simulink model "multi_rotor_sim"  (R2023b)
settings: Solver=ode4  StartTime=0.0  StopTime=inf  FixedStep=ST  RelTol=1e-3
values from neighbouring files (symbols this model uses):
  a0 = 0    [parameters.m]
  ASLOPE = 5.9    [parameters.m]
  Ax = 0.023    [parameters.m]
  Ay = 0.023    [parameters.m]
  Az = 0.106    [parameters.m]
  BLADES = 2    [parameters.m]
  BLCG = 0    [parameters.m]
  BLCP = 0    [parameters.m]
  BLH1 = b*sind(30)    [parameters.m]
  BLH2 = b    (= 0.275)    [parameters.m]
  BLH3 = b*sind(30)    [parameters.m]
  BLH4 = -b*sind(30)    [parameters.m]
  BLH5 = -b    (= -0.275)    [parameters.m]
  BLH6 = -b*sind(30)    [parameters.m]
  chi1 = 1    [parameters.m]
  chi2 = -1    [parameters.m]
  chi3 = 1    [parameters.m]
  chi4 = -1    [parameters.m]
  chi5 = 1    [parameters.m]
  chi6 = -1    [parameters.m]
  CHORD = 17.55e-3    (= 0.01755)    [parameters.m]
  CHORD75 = 21e-3    (= 0.021)    [parameters.m]
  dyn_viscosity = 17.89e-6    (= 1.789e-05)    [parameters.m]
  g0 = 9.80665    [parameters.m]
  href = 0    [parameters.m]
  k_ind = 1.35    [parameters.m]
  k_Omega = 14.92    [parameters.m]
  latref = 44.200626    [parameters.m]
  lonref = 12.063822    [parameters.m]
  m = 2.15    [parameters.m]
  MC_ATT_PITCH = 45*pi/180    (= 0.785398163397)    [parameters.m]
  MC_ATT_ROLL = 45*pi/180    (= 0.785398163397)    [parameters.m]
  MC_PITCH_P = 2    [parameters.m]
  MC_PITCHRATE_D = 0    [parameters.m]
  MC_PITCHRATE_I = 0.05    [parameters.m]
  MC_PITCHRATE_P = 0.09*3    (= 0.27)    [parameters.m]
  MC_RATE_PITCH = 500*pi/180    (= 8.72664625997)    [parameters.m]
  MC_RATE_ROLL = 500*pi/180    (= 8.72664625997)    [parameters.m]
  MC_RATE_YAW = 300*pi/180    (= 5.23598775598)    [parameters.m]
  MC_ROLL_P = 2    [parameters.m]
  MC_ROLLRATE_D = 0    [parameters.m]
  MC_ROLLRATE_I = 0.05    [parameters.m]
  MC_ROLLRATE_P = 0.09*3    (= 0.27)    [parameters.m]
  MC_VEL_FWD = 15    [parameters.m]
  MC_VEL_FWD_OPT = 0.5    [parameters.m]
  MC_VEL_LAT = 15    [parameters.m]
  MC_VEL_LAT_OPT = 0.5    [parameters.m]
  MC_VEL_VERT = 15    [parameters.m]
  MC_YAW_P = 0.55    [parameters.m]
  MC_YAWRATE_D = 0.05    [parameters.m]
  MC_YAWRATE_I = 0.02    [parameters.m]
  MC_YAWRATE_P = 0.15*3    (= 0.45)    [parameters.m]
  MPC_XY_VEL_D_ACC = 0.6    [parameters.m]
  MPC_XY_VEL_I_ACC = 0.8    [parameters.m]
  MPC_XY_VEL_P_ACC = 1.7    [parameters.m]
  MPC_Z_VEL_D_ACC = 0    [parameters.m]
  MPC_Z_VEL_I_ACC = 2    [parameters.m]
  MPC_Z_VEL_P_ACC = 4    [parameters.m]
  n = 0.6359    [parameters.m]
  p00 = 7.145e-2    (= 0.07145)    [parameters.m]
  p01 = 0.4377    [parameters.m]
  p02 = -10.13    [parameters.m]
  p10 = 1.259e-3    (= 0.001259)    [parameters.m]
  p11 = 1.284e-3    (= 0.001284)    [parameters.m]
  p20 = -7.513e-7    (= -7.513e-07)    [parameters.m]
  PWM_hover = (PWM_idle+PWM_max)/2    (= 1550)    [parameters.m]
  PWM_idle = 1100    [parameters.m]
  PWM_max = 2000    [parameters.m]
  ROTOR = 4*0.0254    (= 0.1016)    [parameters.m]
  ST = 0.01    [parameters.m]
  STACG = 0    [parameters.m]
  STACP = 0    [parameters.m]
  STAH1 = -b*cosd(30)    [parameters.m]
  STAH2 = 0    [parameters.m]
  STAH3 = b*cosd(30)    [parameters.m]
  STAH4 = b*cosd(30)    [parameters.m]
  STAH5 = 0    [parameters.m]
  STAH6 = -b*cosd(30)    [parameters.m]
  TERMINAL_SPEED = 0.5    [parameters.m]
  Theta0 = 45*pi/180    (= 0.785398163397)    [parameters.m]
  THETT = -38.0973*pi/180    (= -0.66492332112)    [parameters.m]
  wind_rate = [ 0 0 0 ]'    [parameters.m]
  wind_velocity_e = [ 0 0 0 ]'    [parameters.m]
  WLCG = -0.02    [parameters.m]
  WLCP = -0.08    [parameters.m]
  WLH1 = 32e-3    (= 0.032)    [parameters.m]
  WLH2 = 32e-3    (= 0.032)    [parameters.m]
  WLH3 = 32e-3    (= 0.032)    [parameters.m]
  WLH4 = 32e-3    (= 0.032)    [parameters.m]
  WLH5 = 32e-3    (= 0.032)    [parameters.m]
  WLH6 = 32e-3    (= 0.032)    [parameters.m]
undefined symbols (not defined in the file or in its folder): Earth, WGS84, X, Y, Z
libraries: sm_lib x258, slpidlib x36, nesl_utility x15, sharedtransform x13, aerolibutil x4, aerolibanimutils x3, sharedutil x2, sim3dlib x1, uavsim3dlib x1, shared6dof x1, aerolibtransform2 x1, aerolibatmos2 x1
(part 1 of 11)
settings Model: Creator=Francesco Sessini  LastModifiedBy=fra62

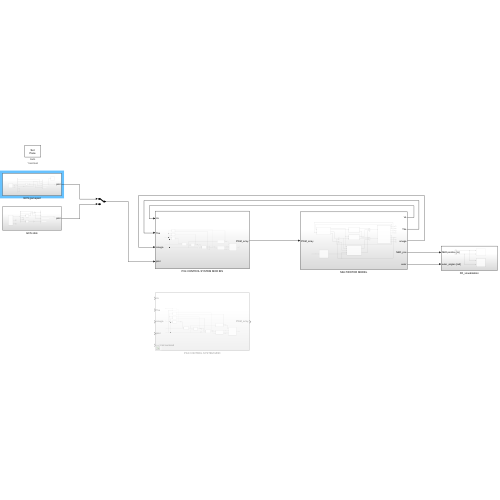
[thumbnail: Simulink's stored preview of the top-level diagram]
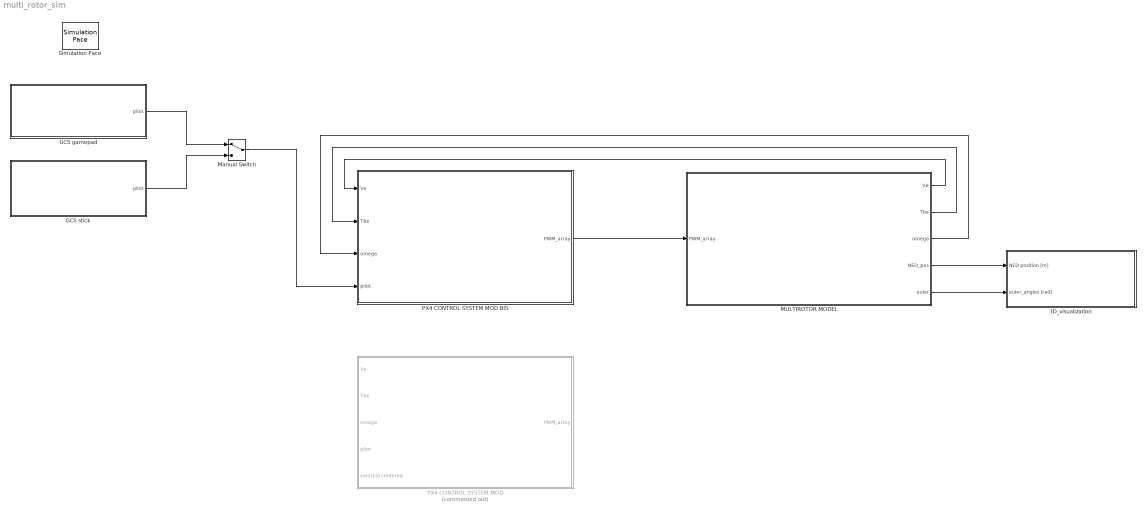
== system multi_rotor_sim ==
  3D_visualization : Subsystem
  GCS gamepad : Subsystem
  GCS stick : Subsystem
  MULTIROTOR MODEL : Subsystem
  Manual Switch : ManualSwitch
  PX4 CONTROL SYSTEM MOD : Subsystem  Commented=on
  PX4 CONTROL SYSTEM MOD BIS : Subsystem
  Simulation Pace : aerolibanimutils/Simulation Pace  SimulationPace=1  SleepMode=Auto  OutputPaceError=off  SampleTime=ST
  wires:
  PX4 CONTROL SYSTEM MOD BIS/1(PWM_array) -> MULTIROTOR MODEL/1(PWM_array)
  MULTIROTOR MODEL/1(Ve) -> PX4 CONTROL SYSTEM MOD BIS/1(Ve)
  MULTIROTOR MODEL/2(Tbe) -> PX4 CONTROL SYSTEM MOD BIS/2(Tbe)
  MULTIROTOR MODEL/3(omega) -> PX4 CONTROL SYSTEM MOD BIS/3(omega)
  Manual Switch/1 -> PX4 CONTROL SYSTEM MOD BIS/4(pilot)
  GCS stick/1(pilot) -> Manual Switch/2
  GCS gamepad/1(pilot) -> Manual Switch/1
  MULTIROTOR MODEL/4(NED_pos) -> 3D_visualization/1(NED position [m])
  MULTIROTOR MODEL/5(euler) -> 3D_visualization/2(euler_angles [rad])

== system multi_rotor_sim/3D_visualization ==
  NED position [m] : Inport
  euler_angles [rad] : Inport  Port=2
  SIMECHANICS 3D SCENE : Subsystem  Commented=on
  UNREAL ENGINE 3D SCENE : Subsystem
  wires:
  NED position [m]/1 -> UNREAL ENGINE 3D SCENE/1(Xe), SIMECHANICS 3D SCENE/1(NED position [m])
  euler_angles [rad]/1 -> UNREAL ENGINE 3D SCENE/2(euler), SIMECHANICS 3D SCENE/2(euler_angles [rad])

== system multi_rotor_sim/GCS gamepad ==
  note: yaw [-1 1] positive right
  note: throttle [-1 1] positive up
  note: pitch [-1 1] positive stick towards pilot
  note: roll [-1 1] positive stick right
  1-D Lookup Table4 : Lookup_n-D  NumberOfTableDimensions=1  BreakpointsForDimension1=[0 1]  Table=[-1 1]  InternalRulePriority=Speed  RndMeth=Simplest
  Demux1 : Demux  Outputs=6
  Display : Display
  Gain1 : Gain  Gain=-1
  Gain5 : Gain  Gain=-1
  Mux1 : Mux
  Pilot Joystick All1 : aerolibanimutils/Pilot Joystick  JoystickID=Joystick1  OutputConfiguration=AllOutputs  SampleTime=ST
      settings: LibrarySourceBlock=aerolibanimutils/Pilot Joystick All
  Terminator{4..7} (4 alike) : Terminator
  pilot : Outport
  wires:
  Gain5/1 -> Mux1/1
  Demux1/1 -> Mux1/2
  Pilot Joystick All1/3 -> Terminator5/1
  Mux1/1 -> Display/1, pilot/1
  Demux1/5 -> Terminator6/1
  Demux1/2 -> Mux1/3
  Pilot Joystick All1/2 -> Terminator4/1
  Demux1/4 -> Gain5/1
  Demux1/3 -> 1-D Lookup Table4/1
  1-D Lookup Table4/1 -> Gain1/1
  Demux1/6 -> Terminator7/1
  Pilot Joystick All1/1 -> Demux1/1
  Gain1/1 -> Mux1/4

== system multi_rotor_sim/GCS stick ==
  note: yaw [-1 1] positive right
  note: roll [-1 1] positive stick right
  note: pitch [-1 1] positive stick towards pilot
  note: throttle [-1 1] positive up
  1-D Lookup Table : Lookup_n-D  NumberOfTableDimensions=1  BreakpointsForDimension1=[0 1]  Table=[-1 1]  InternalRulePriority=Speed  RndMeth=Simplest
  1-D Lookup Table1 : Lookup_n-D  NumberOfTableDimensions=1  BreakpointsForDimension1=[0 1]  Table=[-1 1]  InternalRulePriority=Speed  RndMeth=Simplest
  Demux : Demux  Outputs=6
  Gain : Gain  Gain=-1
  Gain1 : Gain  Gain=-1
  Mux : Mux
  Pilot Joystick All : aerolibanimutils/Pilot Joystick  JoystickID=None  OutputConfiguration=AllOutputs  SampleTime=ST
      settings: LibrarySourceBlock=aerolibanimutils/Pilot Joystick All
  Terminator{,1..3} (4 alike) : Terminator
  pilot : Outport
  wires:
  Demux/2 -> Mux/3
  Pilot Joystick All/2 -> Terminator/1
  Demux/1 -> Mux/2
  1-D Lookup Table1/1 -> Gain1/1
  1-D Lookup Table/1 -> Gain/1
  Demux/3 -> 1-D Lookup Table/1
  Demux/5 -> Terminator3/1
  Demux/6 -> 1-D Lookup Table1/1
  Pilot Joystick All/1 -> Demux/1
  Pilot Joystick All/3 -> Terminator1/1
  Demux/4 -> Terminator2/1
  Gain/1 -> Mux/1
  Mux/1 -> pilot/1
  Gain1/1 -> Mux/4

== system multi_rotor_sim/MULTIROTOR MODEL ==
  PWM_array : Inport
  6DOF (Euler Angles) : shared6dof/6DOF (Euler Angles)  units=Metric (MKS)  mtype=Fixed  rep=Euler Angles  xme_0=Xe_0  Vm_0=V0  eul_0=euler0  pm_0=omega0  mass_0=m  mass_e=0.5  mass_f=2.0  inertia=J  inertia_e=eye(3)  inertia_f=2*eye(3)  k_quat=1.0  vre_flag=on  abi_flag=off  aMode=0  xme_statename=''  Vm_statename=''  eul_statename=''  quat_statename=''  pm_statename=''  mass_statename=''
  Add : Sum  Inputs=+++
  Add1 : Sum  Inputs=+++
  Add2 : Sum  Inputs=-+
  Add3 : Sum  Inputs=-+
  ENVIRONMENT : Subsystem
  ESC+motor : Subsystem
  FRAME DRAG FORCE AND MOMENT : Subsystem
  "GRAVITY FORCE " : Subsystem
  ROTORS FORCE AND MOMENT : Subsystem
  Saturation : Saturate  UpperLimit=PWM_max  LowerLimit=1.1*PWM_idle
  Terminator1 : Terminator
  Terminator2 : Terminator
  Ve : Outport
  Tbe : Outport  Port=2
  omega : Outport  Port=3
  NED_pos : Outport  Port=4
  euler : Outport  Port=5
  wires:
  ESC+motor/1(Omega_array) -> ROTORS FORCE AND MOMENT/5(Omega_array)
  "GRAVITY FORCE "/1(Fgravity) -> Add/1
  "GRAVITY FORCE "/2(Mgravity) -> Add1/1
  6DOF (Euler Angles)/6 -> omega/1, ROTORS FORCE AND MOMENT/4(omega), Add3/2
  Add1/1 -> 6DOF (Euler Angles)/2
  ENVIRONMENT/1(rho) -> ROTORS FORCE AND MOMENT/1(rho), FRAME DRAG FORCE AND MOMENT/1(rho)
  ENVIRONMENT/3(wind_velocity) -> Add2/1
  6DOF (Euler Angles)/2 -> ENVIRONMENT/1(Xe), NED_pos/1
  ENVIRONMENT/4(wind_rate) -> Add3/1
  Add/1 -> 6DOF (Euler Angles)/1
  FRAME DRAG FORCE AND MOMENT/1(F_frame) -> Add/2
  Add3/1 -> ROTORS FORCE AND MOMENT/3(omega_TAS)  "omega_TAS"
  ENVIRONMENT/2(g) -> "GRAVITY FORCE "/1(g)
  Add2/1 -> FRAME DRAG FORCE AND MOMENT/2(TAS), ROTORS FORCE AND MOMENT/2(TAS)  "TAS"
  FRAME DRAG FORCE AND MOMENT/2(M_frame) -> Add1/2
  6DOF (Euler Angles)/5 -> Add2/2
  ROTORS FORCE AND MOMENT/1(Mrotors) -> Add1/3
  6DOF (Euler Angles)/4 -> Tbe/1, ENVIRONMENT/2(Tbe)
  ROTORS FORCE AND MOMENT/2(Frotors) -> Add/3
  6DOF (Euler Angles)/1 -> Ve/1
  6DOF (Euler Angles)/3 -> euler/1
  6DOF (Euler Angles)/7 -> Terminator1/1
  6DOF (Euler Angles)/8 -> Terminator2/1
  PWM_array/1 -> Saturation/1
  Saturation/1 -> ESC+motor/1(PWM_array)

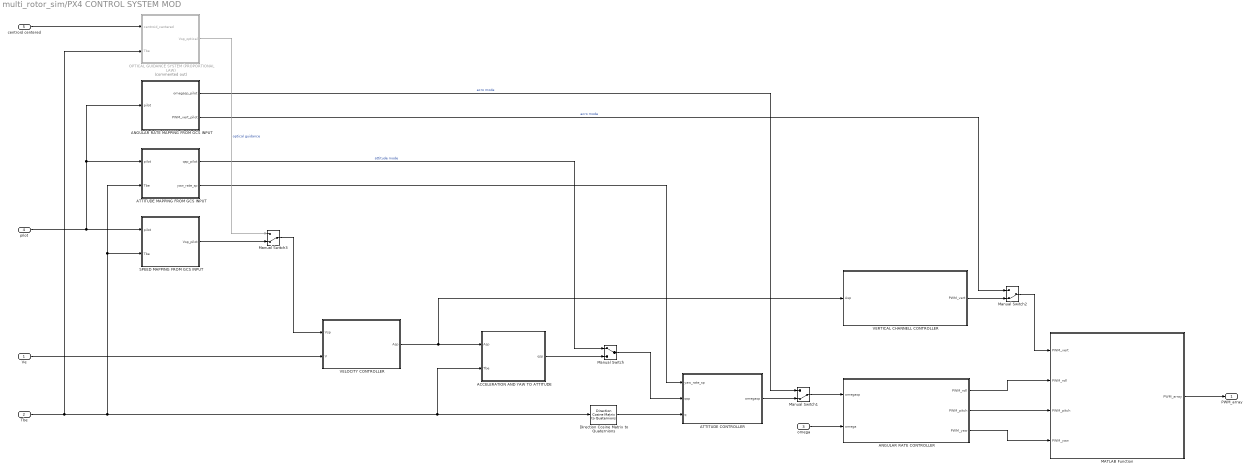
== system multi_rotor_sim/PX4 CONTROL SYSTEM MOD ==
  Ve : Inport
  Tbe : Inport  Port=2
  omega : Inport  Port=3
  pilot : Inport  Port=4
  centroid centered : Inport  Port=5
  ACCELERATION AND YAW TO ATTITUDE : Subsystem
  ANGULAR RATE CONTROLLER : Subsystem
  ANGULAR RATE MAPPING FROM GCS INPUT : Subsystem
  ATTITUDE CONTROLLER : Subsystem
  ATTITUDE MAPPING FROM GCS INPUT : Subsystem
  Direction Cosine Matrix to Quaternions : sharedtransform/Direction Cosine Matrix  to Quaternions  aMode=0  action=None  tolerance=eps(2)
      settings: LibrarySourceBlock=|
      | aerolibtransform2/Direction Cosine Matrix
      | to Quaternions
  MATLAB Function : MATLAB Function  TreatAsAtomicUnit=on
  Manual Switch : ManualSwitch
  Manual Switch1 : ManualSwitch  CurrentSetting=0
  Manual Switch2 : ManualSwitch  CurrentSetting=0
  Manual Switch3 : ManualSwitch  CurrentSetting=0
  OPTICAL GUIDANCE SYSTEM (PROPORTIONAL LAW) : Subsystem  Commented=on
  SPEED MAPPING FROM GCS INPUT : Subsystem
  VELOCITY CONTROLLER : Subsystem
  VERTICAL CHANNELL CONTROLLER : Subsystem
  PWM_array : Outport
  wires:
  ANGULAR RATE CONTROLLER/2(PWM_pitch) -> MATLAB Function/3(PWM_pitch)
  Ve/1 -> VELOCITY CONTROLLER/2(V)
  MATLAB Function/1(PWM_array) -> PWM_array/1
  Tbe/1 -> OPTICAL GUIDANCE SYSTEM (PROPORTIONAL LAW)/2(Tbe), ATTITUDE MAPPING FROM GCS INPUT/2(Tbe), SPEED MAPPING FROM GCS INPUT/2(Tbe), ACCELERATION AND YAW TO ATTITUDE/2(Tbe), Direction Cosine Matrix to Quaternions/1
  VELOCITY CONTROLLER/1(Asp) -> VERTICAL CHANNELL CONTROLLER/1(Asp), ACCELERATION AND YAW TO ATTITUDE/1(Asp)
  omega/1 -> ANGULAR RATE CONTROLLER/2(omega)
  ANGULAR RATE CONTROLLER/1(PWM_roll) -> MATLAB Function/2(PWM_roll)
  ACCELERATION AND YAW TO ATTITUDE/1(qsp) -> Manual Switch/2
  ANGULAR RATE CONTROLLER/3(PWM_yaw) -> MATLAB Function/4(PWM_yaw)
  Direction Cosine Matrix to Quaternions/1 -> ATTITUDE CONTROLLER/3(q)
  Manual Switch/1 -> ATTITUDE CONTROLLER/2(qsp)
  ATTITUDE MAPPING FROM GCS INPUT/1(qsp_pilot) -> Manual Switch/1  "attitude mode"
  pilot/1 -> SPEED MAPPING FROM GCS INPUT/1(pilot), ANGULAR RATE MAPPING FROM GCS INPUT/1(pilot), ATTITUDE MAPPING FROM GCS INPUT/1(pilot)
  ATTITUDE MAPPING FROM GCS INPUT/2(yaw_rate_sp) -> ATTITUDE CONTROLLER/1(yaw_rate_sp)
  ATTITUDE CONTROLLER/1(omegasp) -> Manual Switch1/2
  Manual Switch1/1 -> ANGULAR RATE CONTROLLER/1(omegasp)
  ANGULAR RATE MAPPING FROM GCS INPUT/1(omegasp_pilot) -> Manual Switch1/1  "acro mode"
  VERTICAL CHANNELL CONTROLLER/1(PWM_vert) -> Manual Switch2/2
  Manual Switch2/1 -> MATLAB Function/1(PWM_vert)
  ANGULAR RATE MAPPING FROM GCS INPUT/2(PWM_vert_pilot) -> Manual Switch2/1  "acro mode"
  SPEED MAPPING FROM GCS INPUT/1(Vsp_pilot) -> Manual Switch3/2
  Manual Switch3/1 -> VELOCITY CONTROLLER/1(Vsp)
  OPTICAL GUIDANCE SYSTEM (PROPORTIONAL LAW)/1(Vsp_optical) -> Manual Switch3/1  "optical guidance"
  centroid centered/1 -> OPTICAL GUIDANCE SYSTEM (PROPORTIONAL LAW)/1(centroid_centered)

== system multi_rotor_sim/PX4 CONTROL SYSTEM MOD BIS ==
  Ve : Inport
  Tbe : Inport  Port=2
  omega : Inport  Port=3
  pilot : Inport  Port=4
  ACCELERATION AND YAW TO ATTITUDE : Subsystem
  ANGULAR RATE CONTROLLER : Subsystem
  ANGULAR RATE MAPPING FROM GCS INPUT : Subsystem
  ATTITUDE CONTROLLER : Subsystem
  ATTITUDE MAPPING FROM GCS INPUT : Subsystem
  Direction Cosine Matrix to Quaternions : sharedtransform/Direction Cosine Matrix  to Quaternions  aMode=0  action=None  tolerance=eps(2)
      settings: LibrarySourceBlock=|
      | aerolibtransform2/Direction Cosine Matrix
      | to Quaternions
  MATLAB Function : MATLAB Function  TreatAsAtomicUnit=on
  Manual Switch : ManualSwitch
  Manual Switch1 : ManualSwitch  CurrentSetting=0
  Manual Switch2 : ManualSwitch  CurrentSetting=0
  SPEED MAPPING FROM GCS INPUT : Subsystem
  VELOCITY CONTROLLER : Subsystem
  VERTICAL CHANNELL CONTROLLER : Subsystem
  omega_sp : Mux  Inputs=3
  PWM_array : Outport
  wires:
  ANGULAR RATE CONTROLLER/2(PWM_pitch) -> MATLAB Function/3(PWM_pitch)
  Ve/1 -> VELOCITY CONTROLLER/2(V)
  MATLAB Function/1(PWM_array) -> PWM_array/1
  Tbe/1 -> ATTITUDE MAPPING FROM GCS INPUT/2(Tbe), SPEED MAPPING FROM GCS INPUT/2(Tbe), ACCELERATION AND YAW TO ATTITUDE/2(Tbe), Direction Cosine Matrix to Quaternions/1
  VELOCITY CONTROLLER/1(Asp) -> VERTICAL CHANNELL CONTROLLER/1(Asp), ACCELERATION AND YAW TO ATTITUDE/1(Asp)
  omega/1 -> ANGULAR RATE CONTROLLER/2(omega)
  ANGULAR RATE CONTROLLER/1(PWM_roll) -> MATLAB Function/2(PWM_roll)
  ACCELERATION AND YAW TO ATTITUDE/1(qsp) -> Manual Switch/2
  ANGULAR RATE CONTROLLER/3(PWM_yaw) -> MATLAB Function/4(PWM_yaw)
  Direction Cosine Matrix to Quaternions/1 -> ATTITUDE CONTROLLER/2(q)
  Manual Switch/1 -> ATTITUDE CONTROLLER/1(qsp)
  ATTITUDE MAPPING FROM GCS INPUT/1(qsp_pilot) -> Manual Switch/1  "attitude mode"
  pilot/1 -> SPEED MAPPING FROM GCS INPUT/1(pilot), ANGULAR RATE MAPPING FROM GCS INPUT/1(pilot), ATTITUDE MAPPING FROM GCS INPUT/1(pilot)
  Manual Switch1/1 -> ANGULAR RATE CONTROLLER/1(omegasp)
  ANGULAR RATE MAPPING FROM GCS INPUT/1(omegasp_pilot) -> Manual Switch1/1  "acro mode"
  VERTICAL CHANNELL CONTROLLER/1(PWM_vert) -> Manual Switch2/2
  Manual Switch2/1 -> MATLAB Function/1(PWM_vert)
  ANGULAR RATE MAPPING FROM GCS INPUT/2(PWM_vert_pilot) -> Manual Switch2/1  "acro mode"
  SPEED MAPPING FROM GCS INPUT/1(Vsp_pilot) -> VELOCITY CONTROLLER/1(Vsp)
  ATTITUDE CONTROLLER/1(roll_rate_sp) -> omega_sp/1
  ATTITUDE CONTROLLER/2(pitch_rate_sp) -> omega_sp/2
  omega_sp/1 -> Manual Switch1/2
  ANGULAR RATE MAPPING FROM GCS INPUT/3(yaw_rate_sp_pilot) -> omega_sp/3  "yaw_rate_pilot"

== system multi_rotor_sim/3D_visualization/SIMECHANICS 3D SCENE ==
  NED position [m] : Inport
  euler_angles [rad] : Inport  Port=2
  Constant{1..2,5..8} (6 alike) : Constant  Value=[0 0 0]'
  Constant3 : Constant  Value=0
  Mux : Mux  Inputs=2
  Selector : Selector  InputPortWidth=3  IndexOptions=Index vector (dialog)  Indices=[1 2]  OutputSizes=1
  SimMechanics : Subsystem
  SimMechanics1 : Subsystem
  Simulink - PS converter : Subsystem
  Simulink - PS converter1 : Subsystem
  wires:
  Constant5/1 -> Simulink - PS converter/6(dot^2 eta)
  Selector/1 -> Mux/1
  euler_angles [rad]/1 -> Simulink - PS converter/4(eta)
  NED position [m]/1 -> Selector/1, Simulink - PS converter/2(xi)
  Constant3/1 -> Mux/2
  Constant7/1 -> Simulink - PS converter/3(vi)
  Constant1/1 -> Simulink - PS converter1/3(ai)
  Constant6/1 -> Simulink - PS converter/5(dot eta)
  Mux/1 -> Simulink - PS converter1/1(xi)
  Constant8/1 -> Simulink - PS converter/1(ai)
  Constant2/1 -> Simulink - PS converter1/2(vi)
  connections:
  Simulink - PS converter/RConn1 -- SimMechanics/LConn1
  Simulink - PS converter/RConn2 -- SimMechanics/LConn2
  Simulink - PS converter1/RConn2 -- SimMechanics1/LConn2
  Simulink - PS converter/RConn6 -- SimMechanics/LConn6
  Simulink - PS converter1/RConn1 -- SimMechanics1/LConn1
  Simulink - PS converter1/RConn3 -- SimMechanics1/LConn3
  Simulink - PS converter/RConn3 -- SimMechanics/LConn3
  Simulink - PS converter/RConn4 -- SimMechanics/LConn4
  Simulink - PS converter/RConn5 -- SimMechanics/LConn5

== system multi_rotor_sim/3D_visualization/UNREAL ENGINE 3D SCENE ==
  Xe : Inport
  euler : Inport  Port=2
  Gain : Gain  Gain=diag([1 -1 -1])  Multiplication=Matrix(K*u) (u vector)
  Gain1 : Gain  Gain=diag([-1 -1 1])  Multiplication=Matrix(K*u) (u vector)
  Selector : Selector  InputPortWidth=3  IndexOptions=Index vector (dialog)  Indices=[3 2 1]  OutputSizes=1
  Simulation 3D Scene Configuration : sim3dlib/Simulation 3D Scene Configuration  Priority=0  ProjectFormat=Default Scenes  SceneDesc=US city block  ProjectName=C:\Program Files\MATLAB\R2023b\toolbox\shared\sim3d_projects\automotive_project_windows\UE\WindowsNoEditor\VehicleSimulation.exe  ScenePath=/Game/Maps/USCityBlock  EnableOpenDRIVE=off  vehTagList={'Custom';'Scene Origin';'SimulinkVehicle1'}  vehTag=SimulinkVehicle1  FreeCameraInitialTranslation=[0, 0, 0]  FreeCameraDefaultInitialTranslation=[-6, 0, 2]  FreeCameraInitialRotation=[0, 0, 0]  FreeCameraDefaultInitialRotation=[0, -15, 0]  OpVisEn=off  Ts=0.03  EnableWindow=on  EnableRemoteAccess=off  EnableWeather=off  SunAltitude=40.0  SunAzimuth=90  clouds=10  wind=1  fog=0  rain=0  EnableGeospatial=off  OriginHeight=200  OriginLatitude=40.744652  OriginLongitude=-73.988864  MapStyle=Aerial  AdditionalAssetIDs=[]  UseAdvancedSunSky=off  SolarTime=11  TimeZone=-5  Day=21  Month=9  Year=2022  UseDaylightSavingTime=on  DSTStartDay=10  DSTStartMonth=3  DSTEndDay=3  DSTEndMonth=11  DSTSwitchHour=2  sensorTag=MainCamera1  sensorId=1  sensorName=MainCamera1  mountLoc=Origin  offsetFlag=off  tmountOffset=[0, 0, 0]  rmountOffset=[0, 0, 0]  HorizontalResolution=1280  VerticalResolution=720  HorizontalFOV=60  mountPoint=[0 0 0]  mountOrientation=[0 0 0]  aMode=4  ID=1  GeoTrigger=Inactive
      settings: LibrarySourceBlock=uavsim3dlib/Simulation 3D Scene Configuration
  "Simulation 3D UAV " : uavsim3dlib/Simulation 3D UAV Vehicle  Priority=-1  Mesh=Quadrotor  MeshPath=D:\Documents\MSc_aerospace_eng\unmanned systems\multi-rotor sym\cad_parts  Color=Blue  ActorName=SimulinkVehicle1  UseGlobalFrame=off  InitialTranslation=[0 0 0]  InitialRotation=[0 0 0]  InitialTranslationGlobal=[0 0 0]  InitialGeoOrigin=[0 0 0]  InitialRotationGlobal=[0 0 0]  SampleTime=-1  ActorType=SimulinkVehicle  ID=1  aMode=4  ActorTag=SimulinkVehicle1
  wires:
  Selector/1 -> Gain1/1
  Xe/1 -> Gain/1
  euler/1 -> Selector/1
  Gain1/1 -> "Simulation 3D UAV "/2
  Gain/1 -> "Simulation 3D UAV "/1

== system multi_rotor_sim/MULTIROTOR MODEL/ENVIRONMENT ==
  Xe : Inport
  Tbe : Inport  Port=2
  Constant : Constant  Value=href
  Constant1 : Constant  Value=wind_velocity_e
  Constant2 : Constant  Value=wind_rate
  Flat Earth to LLA : aerolibtransform2/Flat Earth to LLA  units=Metric (MKS)  ptype=Earth (WGS84)  F=1/298.257223563  R=6378137  refPosPort=off  LL0=[latref lonref]  psi=0
  ISA Atmosphere Model : aerolibatmos2/ISA Atmosphere Model  useExtended=off  action=Warning  custom=off  viscosityOut=off  g=9.80665  gamma=1.4  R=287.0531  L=0.0065  h_trop=11000  h_strat=20000  rho0=1.225  P0=101325  T0=288.15  h0=0
  Matrix Multiply : Product  Multiplication=Matrix(*)
  Matrix Multiply1 : Product  Multiplication=Matrix(*)
  Mux : Mux  Inputs=[2 1]
  Reshape : Reshape
  Terminator : Terminator
  Terminator1 : Terminator
  Terminator2 : Terminator
  "WGS84 Gravity Model  " : GravityWGS84
  rho : Outport
  g : Outport  Port=2
  wind_velocity : Outport  Port=3
  wind_rate : Outport  Port=4
  wires:
  "WGS84 Gravity Model  "/1 -> Matrix Multiply/2
  Mux/1 -> Reshape/1
  ISA Atmosphere Model/2 -> Terminator1/1
  Reshape/1 -> "WGS84 Gravity Model  "/1
  Flat Earth to LLA/2 -> ISA Atmosphere Model/1, Mux/2
  Matrix Multiply/1 -> g/1
  Tbe/1 -> Matrix Multiply1/1, Matrix Multiply/1
  ISA Atmosphere Model/4 -> rho/1
  Flat Earth to LLA/1 -> Mux/1
  Constant2/1 -> wind_rate/1
  Constant/1 -> Flat Earth to LLA/2
  Xe/1 -> Flat Earth to LLA/1
  Constant1/1 -> Matrix Multiply1/2
  Matrix Multiply1/1 -> wind_velocity/1
  ISA Atmosphere Model/1 -> Terminator/1
  ISA Atmosphere Model/3 -> Terminator2/1

== system multi_rotor_sim/MULTIROTOR MODEL/ESC+motor ==
  PWM_array : Inport
  Constant : Constant  Value=k_Omega
  Constant1 : Constant  Value=n
  Constant2 : Constant  Value=PWM_idle
  DJI OPTO 3OA + DJI 2212 : MATLAB Function  TreatAsAtomicUnit=on
  Omega_array : Outport
  wires:
  PWM_array/1 -> DJI OPTO 3OA + DJI 2212/4(PWM_array)
  Constant1/1 -> DJI OPTO 3OA + DJI 2212/2(n)
  Constant2/1 -> DJI OPTO 3OA + DJI 2212/3(PWM_idle)
  Constant/1 -> DJI OPTO 3OA + DJI 2212/1(k_Omega)
  DJI OPTO 3OA + DJI 2212/1(Omega_array) -> Omega_array/1

== system multi_rotor_sim/MULTIROTOR MODEL/FRAME DRAG FORCE AND MOMENT ==
  rho : Inport
  TAS : Inport  Port=2
  Constant : Constant  Value=Ax
  Constant1 : Constant  Value=Ay
  Constant2 : Constant  Value=Az
  Constant3 : Constant  Value=STACP
  Constant4 : Constant  Value=BLCP
  Constant5 : Constant  Value=WLCP
  Constant6 : Constant  Value=STACG
  Constant7 : Constant  Value=BLCG
  Constant8 : Constant  Value=WLCG
  FRAME DRAG : MATLAB Function  TreatAsAtomicUnit=on
  F_frame : Outport
  M_frame : Outport  Port=2
  wires:
  TAS/1 -> FRAME DRAG/11(TAS)
  FRAME DRAG/2(M_frame) -> M_frame/1
  Constant7/1 -> FRAME DRAG/8(BLCG)
  rho/1 -> FRAME DRAG/10(rho)
  Constant4/1 -> FRAME DRAG/5(BLCP)
  Constant1/1 -> FRAME DRAG/2(Ay)
  Constant8/1 -> FRAME DRAG/9(WLCG)
  Constant5/1 -> FRAME DRAG/6(WLCP)
  Constant6/1 -> FRAME DRAG/7(STACG)
  Constant/1 -> FRAME DRAG/1(Ax)
  Constant3/1 -> FRAME DRAG/4(STACP)
  FRAME DRAG/1(F_frame) -> F_frame/1
  Constant2/1 -> FRAME DRAG/3(Az)

== system multi_rotor_sim/MULTIROTOR MODEL/GRAVITY FORCE  ==
  g : Inport
  Constant : Constant  Value=zeros(3,1)
  Gain : Gain  Gain=m
  Fgravity : Outport
  Mgravity : Outport  Port=2
  wires:
  g/1 -> Gain/1
  Constant/1 -> Mgravity/1
  Gain/1 -> Fgravity/1

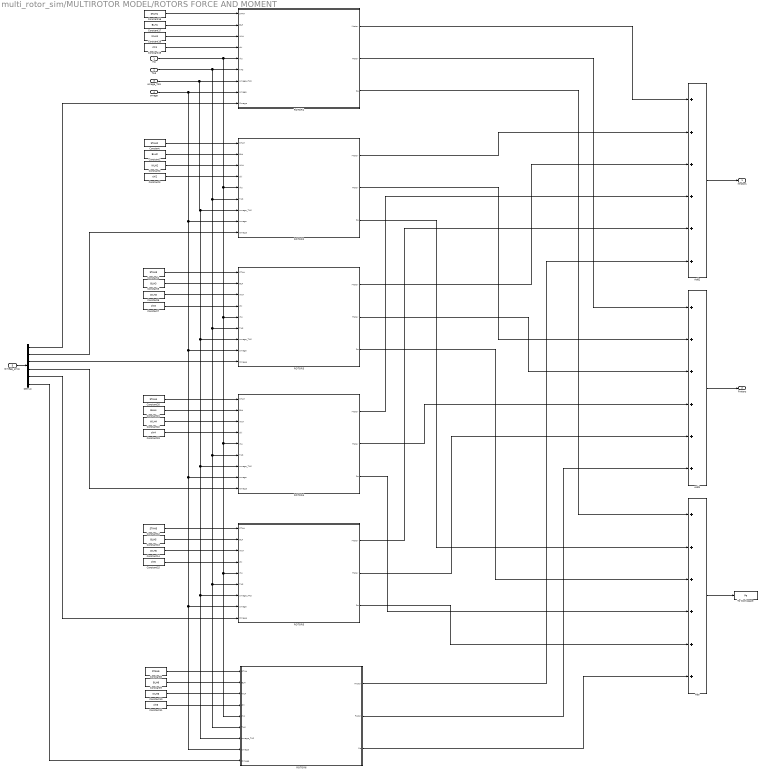
== system multi_rotor_sim/MULTIROTOR MODEL/ROTORS FORCE AND MOMENT ==
  rho : Inport
  TAS : Inport  Port=2
  omega_TAS : Inport  Port=3
  omega : Inport  Port=4
  Omega_array : Inport  Port=5
  Add : Sum  Inputs=++++++
  Add1 : Sum  Inputs=++++++
  Add2 : Sum  Inputs=++++++
  Constant : Constant  Value=STAH2
  Constant1 : Constant  Value=BLH2
  Constant10 : Constant  Value=WLH6
  Constant11 : Constant  Value=chi6
  Constant12 : Constant  Value=STAH5
  Constant13 : Constant  Value=BLH5
  Constant14 : Constant  Value=WLH5
  Constant15 : Constant  Value=chi5
  Constant16 : Constant  Value=STAH1
  Constant17 : Constant  Value=BLH1
  Constant18 : Constant  Value=WLH1
  Constant19 : Constant  Value=chi1
  Constant2 : Constant  Value=WLH2
  Constant20 : Constant  Value=STAH4
  Constant21 : Constant  Value=BLH4
  Constant22 : Constant  Value=WLH4
  Constant23 : Constant  Value=chi4
  Constant3 : Constant  Value=chi2
  Constant4 : Constant  Value=STAH3
  Constant5 : Constant  Value=BLH3
  Constant6 : Constant  Value=WLH3
  Constant7 : Constant  Value=chi3
  Constant8 : Constant  Value=STAH6
  Constant9 : Constant  Value=BLH6
  Demux : Demux  Outputs=6
  ROTOR1 : Subsystem
  ROTOR2 : Subsystem
  ROTOR3 : Subsystem
  ROTOR4 : Subsystem
  ROTOR5 : Subsystem
  ROTOR6 : Subsystem
  To Workspace : ToWorkspace  VariableName=Pe  SampleTime=-1
  Mrotors : Outport
  Frotors : Outport  Port=2
  wires:
  Constant5/1 -> ROTOR3/2(BLH)
  omega/1 -> ROTOR1/8(omega), ROTOR2/8(omega), ROTOR3/8(omega), ROTOR4/8(omega), ROTOR6/8(omega), ROTOR5/8(omega)
  ROTOR4/2(Frotor) -> Add1/4
  omega_TAS/1 -> ROTOR1/7(omega_TAS), ROTOR2/7(omega_TAS), ROTOR3/7(omega_TAS), ROTOR4/7(omega_TAS), ROTOR6/7(omega_TAS), ROTOR5/7(omega_TAS)
  Constant6/1 -> ROTOR3/3(WLH)
  Constant22/1 -> ROTOR4/3(WLH)
  Constant7/1 -> ROTOR3/4(chi)
  Constant15/1 -> ROTOR5/4(chi)
  ROTOR6/3(Pe) -> Add/6
  Add1/1 -> Frotors/1
  ROTOR3/1(Mrotor) -> Add2/3
  Constant4/1 -> ROTOR3/1(STAH)
  Constant21/1 -> ROTOR4/2(BLH)
  Constant9/1 -> ROTOR6/2(BLH)
  ROTOR1/2(Frotor) -> Add1/1
  Constant11/1 -> ROTOR6/4(chi)
  Constant20/1 -> ROTOR4/1(STAH)
  TAS/1 -> ROTOR1/6(TAS), ROTOR2/6(TAS), ROTOR3/6(TAS), ROTOR4/6(TAS), ROTOR6/6(TAS), ROTOR5/6(TAS)
  Constant10/1 -> ROTOR6/3(WLH)
  ROTOR4/1(Mrotor) -> Add2/4
  ROTOR4/3(Pe) -> Add/4
  Constant14/1 -> ROTOR5/3(WLH)
  Constant8/1 -> ROTOR6/1(STAH)
  Add/1 -> To Workspace/1
  Constant2/1 -> ROTOR2/3(WLH)
  Constant19/1 -> ROTOR1/4(chi)
  ROTOR5/1(Mrotor) -> Add2/5
  rho/1 -> ROTOR1/5(rho), ROTOR2/5(rho), ROTOR3/5(rho), ROTOR4/5(rho), ROTOR6/5(rho), ROTOR5/5(rho)
  ROTOR6/1(Mrotor) -> Add2/6
  ROTOR5/2(Frotor) -> Add1/5
  ROTOR2/3(Pe) -> Add/2
  Constant/1 -> ROTOR2/1(STAH)
  Constant18/1 -> ROTOR1/3(WLH)
  Constant3/1 -> ROTOR2/4(chi)
  Constant17/1 -> ROTOR1/2(BLH)
  ROTOR3/3(Pe) -> Add/3
  Constant1/1 -> ROTOR2/2(BLH)
  ROTOR1/1(Mrotor) -> Add2/1
  Constant23/1 -> ROTOR4/4(chi)
  Constant12/1 -> ROTOR5/1(STAH)
  Constant13/1 -> ROTOR5/2(BLH)
  Add2/1 -> Mrotors/1
  ROTOR1/3(Pe) -> Add/1
  Constant16/1 -> ROTOR1/1(STAH)
  ROTOR2/2(Frotor) -> Add1/2
  ROTOR6/2(Frotor) -> Add1/6
  ROTOR3/2(Frotor) -> Add1/3
  ROTOR2/1(Mrotor) -> Add2/2
  ROTOR5/3(Pe) -> Add/5
  Omega_array/1 -> Demux/1
  Demux/1 -> ROTOR1/9(Omega)
  Demux/2 -> ROTOR2/9(Omega)
  Demux/3 -> ROTOR3/9(Omega)
  Demux/4 -> ROTOR4/9(Omega)
  Demux/5 -> ROTOR5/9(Omega)
  Demux/6 -> ROTOR6/9(Omega)

== system multi_rotor_sim/PX4 CONTROL SYSTEM MOD/ACCELERATION AND YAW TO ATTITUDE ==
  Asp : Inport
  Tbe : Inport  Port=2
  Constant : Constant  Value=g0
  Direction Cosine Matrix to Rotation Angles : sharedtransform/Direction Cosine Matrix to Rotation Angles  rotationOrder=ZYX  aMode=aMode  action=None  tolerance=eps(2)
      settings: LibrarySourceBlock=|
      | aerolibtransform2/Direction Cosine Matrix
      | to Rotation Angles
  MATLAB Function : MATLAB Function  TreatAsAtomicUnit=on
  Mux : Mux  Inputs=3
  Rotation Angles to Quaternions : sharedtransform/Rotation Angles to Quaternions  rotationOrder=ZYX  aMode=aMode
  Selector1 : Selector  InputPortWidth=3  IndexOptions=Index vector (dialog)  Indices=[1]  OutputSizes=1
  qsp : Outport
  wires:
  MATLAB Function/1(theta_sp) -> Mux/2
  Selector1/1 -> MATLAB Function/3(psi), Mux/1
  Constant/1 -> MATLAB Function/2(g0)
  Asp/1 -> MATLAB Function/1(Asp)
  MATLAB Function/2(phi_sp) -> Mux/3
  Mux/1 -> Rotation Angles to Quaternions/1
  Rotation Angles to Quaternions/1 -> qsp/1
  Direction Cosine Matrix to Rotation Angles/1 -> Selector1/1
  Tbe/1 -> Direction Cosine Matrix to Rotation Angles/1

== system multi_rotor_sim/PX4 CONTROL SYSTEM MOD/ANGULAR RATE CONTROLLER ==
  omegasp : Inport
  omega : Inport  Port=2
  Gain : Gain  Gain=0.5*(PWM_max-PWM_idle)
  Gain1 : Gain  Gain=0.5*(PWM_max-PWM_idle)
  Gain2 : Gain  Gain=0.5*(PWM_max-PWM_idle)
  PITCHRATE_CONTROLLER : Subsystem
  ROLLRATE_CONTROLLER : Subsystem
  YAWRATE_CONTROLLER : Subsystem
  PWM_roll : Outport
  PWM_pitch : Outport  Port=2
  PWM_yaw : Outport  Port=3
  wires:
  omega/1 -> YAWRATE_CONTROLLER/2(omega), PITCHRATE_CONTROLLER/2(omega), ROLLRATE_CONTROLLER/2(omega)
  ROLLRATE_CONTROLLER/1(delta_roll) -> Gain/1
  omegasp/1 -> YAWRATE_CONTROLLER/1(omegasp), PITCHRATE_CONTROLLER/1(omegasp), ROLLRATE_CONTROLLER/1(omegasp)
  PITCHRATE_CONTROLLER/1(delta_pitch) -> Gain1/1
  YAWRATE_CONTROLLER/1(delta_yaw) -> Gain2/1
  Gain/1 -> PWM_roll/1
  Gain1/1 -> PWM_pitch/1
  Gain2/1 -> PWM_yaw/1

== system multi_rotor_sim/PX4 CONTROL SYSTEM MOD/ANGULAR RATE MAPPING FROM GCS INPUT ==
  pilot : Inport
  Constant1 : Constant  Value=PWM_hover
  Constant2 : Constant  Value=MC_RATE_ROLL
  Constant3 : Constant  Value=MC_RATE_PITCH
  Constant4 : Constant  Value=MC_RATE_YAW
  Gain : Gain  Gain=0.5*(PWM_max-PWM_idle)
  MATLAB Function1 : MATLAB Function  TreatAsAtomicUnit=on
  Sum : Sum  Inputs=|++
  cubic : MATLABFcn  MATLABFcn=u.^3
  omegasp_pilot : Outport
  PWM_vert_pilot : Outport  Port=2
  wires:
  Constant4/1 -> MATLAB Function1/4(MC_RATE_YAW)
  Constant2/1 -> MATLAB Function1/2(MC_RATE_ROLL)
  Constant3/1 -> MATLAB Function1/3(MC_RATE_PITCH)
  MATLAB Function1/1(omegasp_pilot) -> omegasp_pilot/1
  MATLAB Function1/2(delta_throttle) -> Gain/1
  Gain/1 -> Sum/1
  Constant1/1 -> Sum/2
  Sum/1 -> PWM_vert_pilot/1
  pilot/1 -> cubic/1
  cubic/1 -> MATLAB Function1/1(pilot)

== system multi_rotor_sim/PX4 CONTROL SYSTEM MOD/ATTITUDE CONTROLLER ==
  yaw_rate_sp : Inport
  qsp : Inport  Port=2
  q : Inport  Port=3
  Constant : Constant  Value=MC_ROLL_P
  Constant1 : Constant  Value=MC_PITCH_P
  Constant2 : Constant  Value=MC_YAW_P
  MATLAB Function : MATLAB Function  TreatAsAtomicUnit=on
  Quaternion Conjugate : aerolibutil/Quaternion Conjugate
  Quaternion Multiplication : aerolibutil/Quaternion Multiplication
  Quaternion Normalize : sharedutil/Quaternion Normalize  aMode=aMode
  omegasp : Outport
  wires:
  Constant/1 -> MATLAB Function/2(MC_ROLL_P)
  Constant1/1 -> MATLAB Function/3(MC_PITCH_P)
  Constant2/1 -> MATLAB Function/4(MC_YAW_P)
  Quaternion Normalize/1 -> Quaternion Multiplication/1
  Quaternion Multiplication/1 -> MATLAB Function/1(qe)  "qe"
  Quaternion Conjugate/1 -> Quaternion Normalize/1
  qsp/1 -> Quaternion Multiplication/2
  MATLAB Function/1(omegasp) -> omegasp/1
  q/1 -> Quaternion Conjugate/1
  yaw_rate_sp/1 -> MATLAB Function/5(yaw_rate_sp)

== system multi_rotor_sim/PX4 CONTROL SYSTEM MOD/ATTITUDE MAPPING FROM GCS INPUT ==
  pilot : Inport
  Tbe : Inport  Port=2
  Constant2 : Constant  Value=MC_ATT_ROLL
  Constant3 : Constant  Value=MC_ATT_PITCH
  Constant4 : Constant  Value=MC_RATE_YAW
  Direction Cosine Matrix to Rotation Angles : sharedtransform/Direction Cosine Matrix to Rotation Angles  rotationOrder=ZYX  aMode=aMode  action=None  tolerance=eps(2)
      settings: LibrarySourceBlock=|
      | aerolibtransform2/Direction Cosine Matrix
      | to Rotation Angles
  MATLAB Function1 : MATLAB Function  TreatAsAtomicUnit=on
  Matrix Multiply : Product  Multiplication=Matrix(*)
  Rotation Angles to Quaternions : sharedtransform/Rotation Angles to Quaternions  rotationOrder=ZYX  aMode=aMode
  Selector : Selector  InputPortWidth=3  IndexOptions=Index vector (dialog)  Indices=[3 2 1]  OutputSizes=1
  Selector2 : Selector  InputPortWidth=3  IndexOptions=Index vector (dialog)  Indices=[1]  OutputSizes=1
  qsp_pilot : Outport
  yaw_rate_sp : Outport  Port=2
  wires:
  Selector/1 -> Rotation Angles to Quaternions/1
  Constant4/1 -> MATLAB Function1/4(MC_RATE_YAW)
  Constant2/1 -> MATLAB Function1/2(MC_ATT_ROLL)
  Constant3/1 -> MATLAB Function1/3(MC_ATT_PITCH)
  Rotation Angles to Quaternions/1 -> qsp_pilot/1
  pilot/1 -> MATLAB Function1/1(pilot)
  MATLAB Function1/1(eulersp_pilot) -> Selector/1
  Direction Cosine Matrix to Rotation Angles/1 -> Selector2/1
  Selector2/1 -> MATLAB Function1/5(psi)
  Tbe/1 -> Matrix Multiply/1, Direction Cosine Matrix to Rotation Angles/1
  MATLAB Function1/2(yaw_rate_sp) -> Matrix Multiply/2
  Matrix Multiply/1 -> yaw_rate_sp/1

== system multi_rotor_sim/PX4 CONTROL SYSTEM MOD/OPTICAL GUIDANCE SYSTEM (PROPORTIONAL LAW) ==
  centroid_centered : Inport
  Tbe : Inport  Port=2
  Constant2 : Constant  Value=MC_VEL_FWD_OPT
  Constant3 : Constant  Value=MC_VEL_LAT_OPT
  Constant5 : Constant  Value=TERMINAL_SPEED
  Direction Cosine Matrix to Rotation Angles : sharedtransform/Direction Cosine Matrix to Rotation Angles  rotationOrder=ZYX  aMode=aMode  action=None  tolerance=eps(2)
      settings: LibrarySourceBlock=|
      | aerolibtransform2/Direction Cosine Matrix
      | to Rotation Angles
  MATLAB Function : MATLAB Function  TreatAsAtomicUnit=on
  Selector : Selector  InputPortWidth=3  IndexOptions=Index vector (dialog)  Indices=[1 ]  OutputSizes=1
  Vsp_optical : Outport
  wires:
  Constant5/1 -> MATLAB Function/4(TERMINAL_SPEED)
  Direction Cosine Matrix to Rotation Angles/1 -> Selector/1
  MATLAB Function/1(Vsp_optical) -> Vsp_optical/1
  Constant3/1 -> MATLAB Function/3(MC_VEL_LAT)
  centroid_centered/1 -> MATLAB Function/1(centroid_centered)
  Selector/1 -> MATLAB Function/5(psi)
  Constant2/1 -> MATLAB Function/2(MC_VEL_FWD)
  Tbe/1 -> Direction Cosine Matrix to Rotation Angles/1

== system multi_rotor_sim/PX4 CONTROL SYSTEM MOD/SPEED MAPPING FROM GCS INPUT ==
  pilot : Inport
  Tbe : Inport  Port=2
  Constant1 : Constant  Value=MC_VEL_LAT
  Constant2 : Constant  Value=MC_VEL_FWD
  Constant3 : Constant  Value=MC_VEL_VERT
  Direction Cosine Matrix to Rotation Angles : sharedtransform/Direction Cosine Matrix to Rotation Angles  rotationOrder=ZYX  aMode=aMode  action=None  tolerance=eps(2)
      settings: LibrarySourceBlock=|
      | aerolibtransform2/Direction Cosine Matrix
      | to Rotation Angles
  MATLAB Function1 : MATLAB Function  TreatAsAtomicUnit=on
  Selector1 : Selector  InputPortWidth=3  IndexOptions=Index vector (dialog)  Indices=[1]  OutputSizes=1
  Vsp_pilot : Outport
  wires:
  pilot/1 -> MATLAB Function1/1(pilot)
  Constant1/1 -> MATLAB Function1/4(MC_VEL_LAT)
  Constant2/1 -> MATLAB Function1/3(MC_VEL_FWD)
  Constant3/1 -> MATLAB Function1/5(MC_VEL_VERT)
  Tbe/1 -> Direction Cosine Matrix to Rotation Angles/1
  Direction Cosine Matrix to Rotation Angles/1 -> Selector1/1
  MATLAB Function1/1(Vsp_pilot_inertial) -> Vsp_pilot/1
  Selector1/1 -> MATLAB Function1/2(psi)

== system multi_rotor_sim/PX4 CONTROL SYSTEM MOD/VELOCITY CONTROLLER ==
  Vsp : Inport
  V : Inport  Port=2
  Mux : Mux  Inputs=3
  X_SPEED_CONTROLLER : Subsystem
  Y_SPEED_CONTROLLER : Subsystem
  Z_SPEED_CONTROLLER : Subsystem
  Asp : Outport
  wires:
  V/1 -> Z_SPEED_CONTROLLER/2(V), Y_SPEED_CONTROLLER/2(V), X_SPEED_CONTROLLER/2(V)
  X_SPEED_CONTROLLER/1(Asp_x) -> Mux/1
  Vsp/1 -> Z_SPEED_CONTROLLER/1(Vsp), Y_SPEED_CONTROLLER/1(Vsp), X_SPEED_CONTROLLER/1(Vsp)
  Mux/1 -> Asp/1
  Y_SPEED_CONTROLLER/1(Asp_y) -> Mux/2
  Z_SPEED_CONTROLLER/1(Asp_z) -> Mux/3

== system multi_rotor_sim/PX4 CONTROL SYSTEM MOD/VERTICAL CHANNELL CONTROLLER ==
  Asp : Inport
  Constant : Constant  Value=g0
  Constant1 : Constant  Value=PWM_hover
  Gain : Gain  Gain=0.5*(PWM_max-PWM_idle)
  MATLAB Function : MATLAB Function  TreatAsAtomicUnit=on
  Saturation : Saturate  UpperLimit=1  LowerLimit=-1
  Sum : Sum  Inputs=|++
  PWM_vert : Outport
  wires:
  Constant/1 -> MATLAB Function/2(g0)
  Asp/1 -> MATLAB Function/1(Asp)
  MATLAB Function/1(delta_vert) -> Saturation/1
  Saturation/1 -> Gain/1
  Gain/1 -> Sum/1
  Sum/1 -> PWM_vert/1
  Constant1/1 -> Sum/2

== system multi_rotor_sim/PX4 CONTROL SYSTEM MOD BIS/ACCELERATION AND YAW TO ATTITUDE ==
  Asp : Inport
  Tbe : Inport  Port=2
  Constant : Constant  Value=g0
  Direction Cosine Matrix to Rotation Angles : sharedtransform/Direction Cosine Matrix to Rotation Angles  rotationOrder=ZYX  aMode=aMode  action=None  tolerance=eps(2)
      settings: LibrarySourceBlock=|
      | aerolibtransform2/Direction Cosine Matrix
      | to Rotation Angles
  MATLAB Function : MATLAB Function  TreatAsAtomicUnit=on
  Mux : Mux  Inputs=3
  Rotation Angles to Quaternions : sharedtransform/Rotation Angles to Quaternions  rotationOrder=ZYX  aMode=aMode
  Selector1 : Selector  InputPortWidth=3  IndexOptions=Index vector (dialog)  Indices=[1]  OutputSizes=1
  qsp : Outport
  wires:
  MATLAB Function/1(theta_sp) -> Mux/2
  Selector1/1 -> MATLAB Function/3(psi), Mux/1
  Constant/1 -> MATLAB Function/2(g0)
  Asp/1 -> MATLAB Function/1(Asp)
  MATLAB Function/2(phi_sp) -> Mux/3
  Mux/1 -> Rotation Angles to Quaternions/1
  Rotation Angles to Quaternions/1 -> qsp/1
  Direction Cosine Matrix to Rotation Angles/1 -> Selector1/1
  Tbe/1 -> Direction Cosine Matrix to Rotation Angles/1

== system multi_rotor_sim/PX4 CONTROL SYSTEM MOD BIS/ANGULAR RATE CONTROLLER ==
  omegasp : Inport
  omega : Inport  Port=2
  Gain : Gain  Gain=0.5*(PWM_max-PWM_idle)
  Gain1 : Gain  Gain=0.5*(PWM_max-PWM_idle)
  Gain2 : Gain  Gain=0.5*(PWM_max-PWM_idle)
  PITCHRATE_CONTROLLER : Subsystem
  ROLLRATE_CONTROLLER : Subsystem
  YAWRATE_CONTROLLER : Subsystem
  PWM_roll : Outport
  PWM_pitch : Outport  Port=2
  PWM_yaw : Outport  Port=3
  wires:
  omega/1 -> YAWRATE_CONTROLLER/2(omega), PITCHRATE_CONTROLLER/2(omega), ROLLRATE_CONTROLLER/2(omega)
  ROLLRATE_CONTROLLER/1(delta_roll) -> Gain/1
  omegasp/1 -> YAWRATE_CONTROLLER/1(omegasp), PITCHRATE_CONTROLLER/1(omegasp), ROLLRATE_CONTROLLER/1(omegasp)
  PITCHRATE_CONTROLLER/1(delta_pitch) -> Gain1/1
  YAWRATE_CONTROLLER/1(delta_yaw) -> Gain2/1
  Gain/1 -> PWM_roll/1
  Gain1/1 -> PWM_pitch/1
  Gain2/1 -> PWM_yaw/1

== system multi_rotor_sim/PX4 CONTROL SYSTEM MOD BIS/ANGULAR RATE MAPPING FROM GCS INPUT ==
  pilot : Inport
  Constant1 : Constant  Value=PWM_hover
  Constant2 : Constant  Value=MC_RATE_ROLL
  Constant3 : Constant  Value=MC_RATE_PITCH
  Constant4 : Constant  Value=MC_RATE_YAW
  Gain : Gain  Gain=0.5*(PWM_max-PWM_idle)
  MATLAB Function1 : MATLAB Function  TreatAsAtomicUnit=on
  Selector : Selector  InputPortWidth=3  IndexOptions=Index vector (dialog)  Indices=[3]  OutputSizes=1
  Sum : Sum  Inputs=|++
  cubic : MATLABFcn  MATLABFcn=u.^3
  omegasp_pilot : Outport
  PWM_vert_pilot : Outport  Port=2
  yaw_rate_sp_pilot : Outport  Port=3
  wires:
  Constant4/1 -> MATLAB Function1/4(MC_RATE_YAW)
  Constant2/1 -> MATLAB Function1/2(MC_RATE_ROLL)
  Constant3/1 -> MATLAB Function1/3(MC_RATE_PITCH)
  MATLAB Function1/1(omegasp_pilot) -> Selector/1, omegasp_pilot/1
  MATLAB Function1/2(delta_throttle) -> Gain/1
  Gain/1 -> Sum/1
  Constant1/1 -> Sum/2
  Sum/1 -> PWM_vert_pilot/1
  pilot/1 -> cubic/1
  cubic/1 -> MATLAB Function1/1(pilot)
  Selector/1 -> yaw_rate_sp_pilot/1

== system multi_rotor_sim/PX4 CONTROL SYSTEM MOD BIS/ATTITUDE CONTROLLER ==
  qsp : Inport
  q : Inport  Port=2
  Constant : Constant  Value=MC_ROLL_P
  Constant1 : Constant  Value=MC_PITCH_P
  Constant2 : Constant  Value=MC_YAW_P
  Demux : Demux  Outputs=3
  MATLAB Function : MATLAB Function  TreatAsAtomicUnit=on
  Quaternion Conjugate : aerolibutil/Quaternion Conjugate
  Quaternion Multiplication : aerolibutil/Quaternion Multiplication
  Quaternion Normalize : sharedutil/Quaternion Normalize  aMode=aMode
  Terminator : Terminator
  roll_rate_sp : Outport
  pitch_rate_sp : Outport  Port=2
  wires:
  Constant/1 -> MATLAB Function/2(MC_ROLL_P)
  Constant1/1 -> MATLAB Function/3(MC_PITCH_P)
  Constant2/1 -> MATLAB Function/4(MC_YAW_P)
  Quaternion Normalize/1 -> Quaternion Multiplication/1
  Quaternion Multiplication/1 -> MATLAB Function/1(qe)  "qe"
  Quaternion Conjugate/1 -> Quaternion Normalize/1
  qsp/1 -> Quaternion Multiplication/2
  q/1 -> Quaternion Conjugate/1
  MATLAB Function/1(omegasp) -> Demux/1
  Demux/1 -> roll_rate_sp/1
  Demux/2 -> pitch_rate_sp/1
  Demux/3 -> Terminator/1

== system multi_rotor_sim/PX4 CONTROL SYSTEM MOD BIS/ATTITUDE MAPPING FROM GCS INPUT ==
  pilot : Inport
  Tbe : Inport  Port=2
  Constant2 : Constant  Value=MC_ATT_ROLL
  Constant3 : Constant  Value=MC_ATT_PITCH
  Direction Cosine Matrix to Rotation Angles : sharedtransform/Direction Cosine Matrix to Rotation Angles  rotationOrder=ZYX  aMode=aMode  action=None  tolerance=eps(2)
      settings: LibrarySourceBlock=|
      | aerolibtransform2/Direction Cosine Matrix
      | to Rotation Angles
  MATLAB Function1 : MATLAB Function  TreatAsAtomicUnit=on
  Rotation Angles to Quaternions : sharedtransform/Rotation Angles to Quaternions  rotationOrder=ZYX  aMode=aMode
  Selector : Selector  InputPortWidth=3  IndexOptions=Index vector (dialog)  Indices=[3 2 1]  OutputSizes=1
  Selector2 : Selector  InputPortWidth=3  IndexOptions=Index vector (dialog)  Indices=[1]  OutputSizes=1
  qsp_pilot : Outport
  wires:
  Selector/1 -> Rotation Angles to Quaternions/1
  Constant2/1 -> MATLAB Function1/2(MC_ATT_ROLL)
  Constant3/1 -> MATLAB Function1/3(MC_ATT_PITCH)
  Rotation Angles to Quaternions/1 -> qsp_pilot/1
  pilot/1 -> MATLAB Function1/1(pilot)
  MATLAB Function1/1(eulersp_pilot) -> Selector/1
  Direction Cosine Matrix to Rotation Angles/1 -> Selector2/1
  Selector2/1 -> MATLAB Function1/4(psi)
  Tbe/1 -> Direction Cosine Matrix to Rotation Angles/1

== system multi_rotor_sim/PX4 CONTROL SYSTEM MOD BIS/SPEED MAPPING FROM GCS INPUT ==
  pilot : Inport
  Tbe : Inport  Port=2
  Constant1 : Constant  Value=MC_VEL_LAT
  Constant2 : Constant  Value=MC_VEL_FWD
  Constant3 : Constant  Value=MC_VEL_VERT
  Direction Cosine Matrix to Rotation Angles : sharedtransform/Direction Cosine Matrix to Rotation Angles  rotationOrder=ZYX  aMode=aMode  action=None  tolerance=eps(2)
      settings: LibrarySourceBlock=|
      | aerolibtransform2/Direction Cosine Matrix
      | to Rotation Angles
  MATLAB Function1 : MATLAB Function  TreatAsAtomicUnit=on
  Selector1 : Selector  InputPortWidth=3  IndexOptions=Index vector (dialog)  Indices=[1]  OutputSizes=1
  Vsp_pilot : Outport
  wires:
  pilot/1 -> MATLAB Function1/1(pilot)
  Constant1/1 -> MATLAB Function1/4(MC_VEL_LAT)
  Constant2/1 -> MATLAB Function1/3(MC_VEL_FWD)
  Constant3/1 -> MATLAB Function1/5(MC_VEL_VERT)
  Tbe/1 -> Direction Cosine Matrix to Rotation Angles/1
  Direction Cosine Matrix to Rotation Angles/1 -> Selector1/1
  MATLAB Function1/1(Vsp_pilot_inertial) -> Vsp_pilot/1
  Selector1/1 -> MATLAB Function1/2(psi)

== system multi_rotor_sim/PX4 CONTROL SYSTEM MOD BIS/VELOCITY CONTROLLER ==
  Vsp : Inport
  V : Inport  Port=2
  Mux : Mux  Inputs=3
  X_SPEED_CONTROLLER : Subsystem
  Y_SPEED_CONTROLLER : Subsystem
  Z_SPEED_CONTROLLER : Subsystem
  Asp : Outport
  wires:
  V/1 -> Z_SPEED_CONTROLLER/2(V), Y_SPEED_CONTROLLER/2(V), X_SPEED_CONTROLLER/2(V)
  X_SPEED_CONTROLLER/1(Asp_x) -> Mux/1
  Vsp/1 -> Z_SPEED_CONTROLLER/1(Vsp), Y_SPEED_CONTROLLER/1(Vsp), X_SPEED_CONTROLLER/1(Vsp)
  Mux/1 -> Asp/1
  Y_SPEED_CONTROLLER/1(Asp_y) -> Mux/2
  Z_SPEED_CONTROLLER/1(Asp_z) -> Mux/3

== system multi_rotor_sim/PX4 CONTROL SYSTEM MOD BIS/VERTICAL CHANNELL CONTROLLER ==
  Asp : Inport
  Constant : Constant  Value=g0
  Constant1 : Constant  Value=PWM_hover
  Gain : Gain  Gain=0.5*(PWM_max-PWM_idle)
  MATLAB Function : MATLAB Function  TreatAsAtomicUnit=on
  Saturation : Saturate  UpperLimit=1  LowerLimit=-1
  Sum : Sum  Inputs=|++
  PWM_vert : Outport
  wires:
  Constant/1 -> MATLAB Function/2(g0)
  Asp/1 -> MATLAB Function/1(Asp)
  MATLAB Function/1(delta_vert) -> Saturation/1
  Saturation/1 -> Gain/1
  Gain/1 -> Sum/1
  Sum/1 -> PWM_vert/1
  Constant1/1 -> Sum/2
